simulink model "MSE452_Wind_Project_Model_Student_R2018b"  (R2023a)
settings: Solver=ode45  StartTime=0.0  StopTime=0.4  MaxStep=1e-5  RelTol=1e-3
values from neighbouring files (symbols this model uses):
  Cdc_wind = Cb_wind*3    [MSE452_Wind_Project_Model_Parameters_Student.m]
  Cin = 0.12*Cb_wind    [MSE452_Wind_Project_Model_Parameters_Student.m]
  Fb = 60    [MSE452_Wind_Project_Model_Parameters_Student.m]
  Fs_inv_wind = 3000    [MSE452_Wind_Project_Model_Parameters_Student.m]
  Fsampling = 10e3    (= 10000)    [MSE452_Wind_Project_Model_Parameters_Student.m]
  Ib_wind = Sb_wind/(3*Vb)    [MSE452_Wind_Project_Model_Parameters_Student.m]
  J = 2*H*Sb_wind/(Omega_gen_b^2)    (= 106.875544898)    [MSE452_Wind_Project_Model_Parameters_Student.m]
  Lboost_wind = 0.5*Lb_wind    [MSE452_Wind_Project_Model_Parameters_Student.m]
  Ld = 0.5*Lb_wind    [MSE452_Wind_Project_Model_Parameters_Student.m]
  Lgrid_pu_wind = 0.005    [MSE452_Wind_Project_Model_Parameters_Student.m]
  Lgrid_wind = 0.2*Lb_wind    [MSE452_Wind_Project_Model_Parameters_Student.m]
  Lq = 0.5*Lb_wind    [MSE452_Wind_Project_Model_Parameters_Student.m]
  Omega_gen_b = 2*pi*53.33    (= 335.082272432)    [MSE452_Wind_Project_Model_Parameters_Student.m]
  Ppairs = 16    [MSE452_Wind_Project_Model_Parameters_Student.m]
  Rgrid_wind = Rgrid_pu*Zb_wind    [MSE452_Wind_Project_Model_Parameters_Student.m]
  Rs = 0.01*Zb_wind    [MSE452_Wind_Project_Model_Parameters_Student.m]
  Tb = Ppairs*Sb_wind/Omega_gen_b    (= 71624.2009039)    [MSE452_Wind_Project_Model_Parameters_Student.m]
  Vb = 690/sqrt(3)    [MSE452_Wind_Project_Model_Parameters_Student.m]
  Vdc_ref_wind = sqrt(6)/ma    [MSE452_Wind_Project_Model_Parameters_Student.m]
  Wind_speed_b = 12    [MSE452_Wind_Project_Model_Parameters_Student.m]
undefined symbols (not defined in the file or in its folder): Rdc
libraries: spsCurrentMeasurementLib x11, spsVoltageMeasurementLib x8, spsSeriesRLCBranchLib x3, powerlib_extras x3, simulink x3, spsControlledVoltageSourceLib x2, spsUniversalBridgeLib x2, simulink_extras x2, spsThreePhaseSeriesRLCBranchLib x1, spsPermanentMagnetSynchronousMachineLib x1, spsPower3phInstantaneousLib x1, slpidlib x1
settings Model: Creator=Student  LastModifiedBy=auamai
settings SolverCC: ZeroCrossAlgorithm=Adaptive  AlgebraicLoopSolver=TrustRegion
settings DataIOCC: ReturnWorkspaceOutputs=off
settings OptimizationCC: LifeSpan=inf
settings DebuggingCC: UnconnectedInputMsg=warning  UnconnectedOutputMsg=warning  UnconnectedLineMsg=warning  ArithmeticOperatorsInVariantConditions=warning
settings HardwareCC: ProdBitPerSizeT=32  ProdBitPerPtrDiffT=32  ProdWordSize=32  ProdHWDeviceType=Specified
settings ModelReferenceCC: EnableRefExpFcnMdlSchedulingChecks=on
settings SFSimCC: SimUseLocalCustomCode=off  CustomCodeUndefinedFunction=UseInterfaceOnly
settings RTWCC: RTWUseLocalCustomCode=off
settings CodeAppCC: StateflowObjectComments=on
settings SimscapeCC: SimscapeNormalizeSystem=off

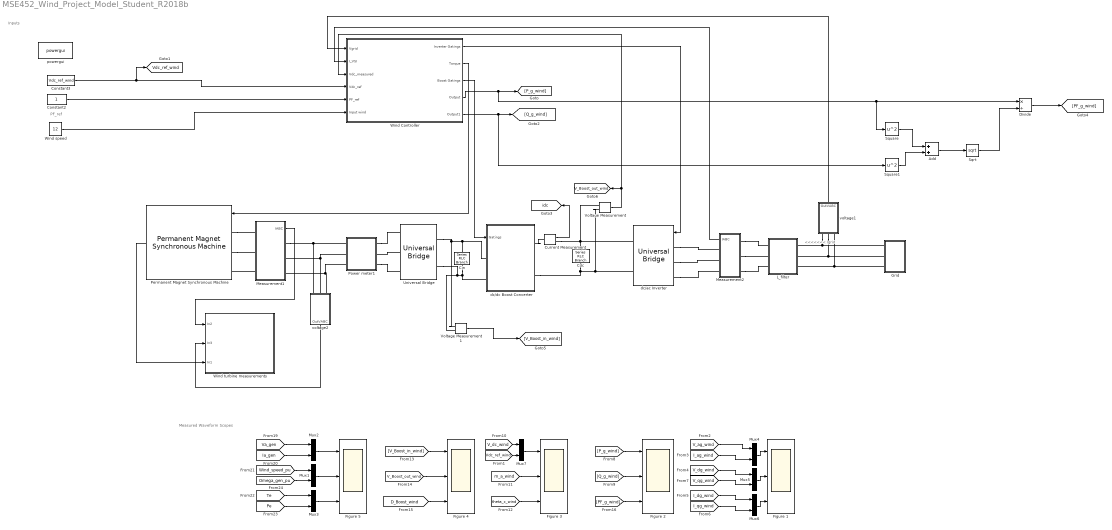
== system MSE452_Wind_Project_Model_Student_R2018b ==
  note: PF_ref
  note: Inputs
  note: <<<<<<< Igrid
  note: Measured Waveform Scopes
  " voltage1" : Subsystem  mask{Base=Vb}
      mask prompts: Base "Base value"
  " voltage2" : Subsystem  mask{Base=Vb}
      mask prompts: Base "Base value"
  Add : Sum
  Cdc : spsSeriesRLCBranchLib/Series RLC Branch  LConnTagsString=__new0  RConnTagsString=__new0  BranchType=C  Resistance=1e-4  Inductance=200e-6  SetiL0=off  InitialCurrent=0  Capacitance=Cdc_wind  Setx0=on  InitialVoltage=Vdc_capacitor_initial_wind  Measurements=None
  Cin : spsSeriesRLCBranchLib/Series RLC Branch  LConnTagsString=__new0  RConnTagsString=__new0  BranchType=C  Resistance=Rdc  Inductance=1e-3  SetiL0=off  InitialCurrent=0  Capacitance=Cin  Setx0=off  InitialVoltage=Vdc_capacitor_initial  Measurements=None
  Constant2 : Constant
  Constant3 : Constant  Value=Vdc_ref_wind
  Current Measurement : spsCurrentMeasurementLib/Current Measurement  PhasorSimulation=off  OutputType=Complex  PSBequivalent=0
  Divide : Product  Inputs=*/
  Figure {1..5} (5 alike) : Scope  NumInputPorts=3
  Grid : Subsystem
  L_filter : Subsystem
  Measurement1 : Subsystem  mask{Base=Ib_wind}
      mask prompts: Base "Base value"
  Measurement2 : Subsystem  mask{Base=Ib_wind}
      mask prompts: Base "Base value"
  Mux{1..7} (7 alike) : Mux  Inputs=2
  Permanent Magnet Synchronous Machine : spsPermanentMagnetSynchronousMachineLib/Permanent Magnet Synchronous Machine  NbPhases=3  FluxDistribution=Sinusoidal  RotorType=Salient-pole  MechanicalLoad=Torque Tm  PresetModel=No  ShowDetailedParameters=on  MeasurementBus=off  Resistance=Rs  Inductance=8.5e-3  dqInductances=[Ld, Lq]  La=0.000395  MachineConstant=Voltage Constant (V_peak L-L / krpm)  Flux=1.6813  VoltageCst=sqrt(2)*Vb*sqrt(3)*(1000/((Omega_gen_b/2/pi)*60/Ppairs))  TorqueCst=40.3518  Flat=120  Mechanical=[J 0.0004924 Ppairs 0]  PolePairs=4  InitialConditions=[15, 0, 0, 0]  InitialConditions5ph=[0 0 0 0 0 0]  RefAngle=Aligned with phase A axis (original Park)  IterativeDiscreteModel=Trapezoidal non iterative  TsBlock=-1  TsPowergui=0
  Power meter1 : Subsystem
  Sqrt : Sqrt
  Square : Math  Operator=square
  Square1 : Math  Operator=square
  Universal Bridge : spsUniversalBridgeLib/Universal Bridge  Arms=3  SnubberResistance=1e5  SnubberCapacitance=inf  Device=Diodes  Ron=1e-3  Lon=0  ForwardVoltages="[  0  0  ]"  ForwardVoltage=0  GTOparameters=[ 10e-6 , 20e-6 ]  IGBTparameters=[ 1e-6 , 2e-6 ]  Measurements=None  Measurements_2=None  converterType=Rectifier
  Voltage Measurement : spsVoltageMeasurementLib/Voltage Measurement  PhasorSimulation=off  OutputType=Complex  PSBequivalent=0
  Voltage Measurement1 : spsVoltageMeasurementLib/Voltage Measurement  PhasorSimulation=off  OutputType=Complex  PSBequivalent=0
  Wind Controller : Subsystem
  Wind speed : Constant  Value=12
  Wind turbine measurements : Subsystem
  dc/ac Inverter : spsUniversalBridgeLib/Universal Bridge  Arms=3  SnubberResistance=1e5  SnubberCapacitance=inf  Device=IGBT / Diodes  Ron=1e-6  Lon=0  ForwardVoltages="[  0  0  ]"  ForwardVoltage=0  GTOparameters=[ 10e-6 , 20e-6 ]  IGBTparameters=[ 1e-6 , 2e-6 ]  Measurements=None  Measurements_2=None  converterType=Rectifier
  dc/dc Boost Converter : Subsystem
  powergui : sps_lib/powergui  Priority=1  SimulationMode=Discrete  SampleTime=1e-6  frequency=60  Iterations=50  frequencyindice=0  Pbase=100e6  ErrMax=1e-4  UnitsV=kV  UnitsW=MW  buscounter=0  FunctionMessages=off  echomessages=off  EnableUseOfTLC=off  CurrentSourceSwitches=off  DisableSnubberDevices=off  DisableRonSwitches=off  DisableVfSwitches=off  DisplayEquations=off  AutomaticDiscreteSolvers=off  SolverType=Tustin/Backward Euler (TBE)  Interpol=off  ExternalGateDelay=off  methode=off  Ts=100  x0status=blocks  SPID=on  SwTol=0  HookPort=off  NonlinearTolerance=1e-4  nMaxIteration=100  ContinueOnMaxIteration=off  RestoreLinks=warning  ResistiveCurrentMeasurement=off  Frange=[0:2:500]  Ylog=off  Xlog=on  ShowGrid=off  save=off  variable=ZData  structure=0  ZoomFFT=off  StartTime=0.0  cycles=1  DisplayStyle=1  fundamental=60  FreqAxis=off  MaxFrequency=1000  frequencyindicesteady=1  RmsSteady=1  display=off
  tag scope: V_Boost_out_wind=global, Vdc_ref_wind=global, idc=global
  wires:
  [V_Boost_in_wind] -> Figure 4/1
  [Omega_gen_pu] -> Mux1/2
  [I_dg_wind] -> Mux6/1
  [Va_gen] -> Mux2/1
  Measurement2/1(IABC) -> Wind Controller/2(I_VSI)
  [Wind_speed_pu] -> Mux1/1
  [V_qg_wind] -> Mux5/2
  [m_a_wind] -> Figure 3/2
  [D_Boost_wind] -> Figure 4/3
  [V_Boost_out_wind] -> Figure 4/2
  Current Measurement/1 -> [idc]
  [I_ag_wind] -> Mux4/2
  Wind Controller/1(Inverter Gatings) -> dc/ac Inverter/1
  [Te] -> Mux3/1
  Voltage Measurement/1 -> Wind Controller/3(Vdc_measured), [V_Boost_out_wind]
  Voltage Measurement1/1 -> [V_Boost_in_wind]
  [V_dg_wind] -> Mux5/1
  " voltage1"/1(OutVABC) -> Wind Controller/1(Vgrid)
  [P_g_wind] -> Figure 2/1
  Mux2/1 -> Figure 5/1
  [theta_c_wind] -> Figure 3/3
  [Pe] -> Mux3/2
  [I_qg_wind] -> Mux6/2
  [Ia_gen] -> Mux2/2
  [V_ag_wind] -> Mux4/1
  [Q_g_wind] -> Figure 2/2
  [PF_g_wind] -> Figure 2/3
  Mux1/1 -> Figure 5/2
  Mux3/1 -> Figure 5/3
  Constant2/1 -> Wind Controller/5(PF_ref)
  Wind speed/1 -> Wind Controller/6(Input wind)
  Wind Controller/2(Torque) -> Permanent Magnet Synchronous Machine/1
  Permanent Magnet Synchronous Machine/1 -> Wind turbine measurements/3(In1)
  Measurement1/1(IABC) -> Wind turbine measurements/1(In2)
  " voltage2"/1(OutVABC) -> Wind turbine measurements/2(In3)
  Constant3/1 -> [Vdc_ref_wind], Wind Controller/4(Vdc_ref)
  Wind Controller/3(Boost Gatings) -> dc/dc Boost Converter/1(Gatings)
  Mux7/1 -> Figure 3/1
  [V_dc_wind] -> Mux7/1
  [Vdc_ref_wind] -> Mux7/2
  Wind Controller/4(Output) -> Square/1, Divide/1, [P_g_wind]
  Wind Controller/5(Output1) -> Square1/1, [Q_g_wind]
  Square/1 -> Add/1
  Square1/1 -> Add/2
  Add/1 -> Sqrt/1
  Sqrt/1 -> Divide/2
  Divide/1 -> [PF_g_wind]
  Mux6/1 -> Figure 1/3
  Mux5/1 -> Figure 1/2
  Mux4/1 -> Figure 1/1
  connections:
  dc/dc Boost Converter/LConn1 -- Voltage Measurement1/LConn1 -- Universal Bridge/RConn1 -- Cin/LConn1
  Cdc/LConn1 -- Current Measurement/RConn1 -- dc/ac Inverter/RConn1 -- Voltage Measurement/LConn1
  Voltage Measurement/LConn2 -- Cdc/RConn1 -- dc/dc Boost Converter/RConn2 -- dc/ac Inverter/RConn2
  Voltage Measurement1/LConn2 -- Universal Bridge/RConn2 -- Cin/RConn1 -- dc/dc Boost Converter/LConn2
  Measurement1/RConn1 -- Power meter1/LConn1 -- " voltage2"/LConn1
  " voltage2"/LConn3 -- Power meter1/LConn3 -- Measurement1/RConn3
  " voltage2"/LConn2 -- Power meter1/LConn2 -- Measurement1/RConn2
  Permanent Magnet Synchronous Machine/LConn1 -- Measurement1/LConn1
  Permanent Magnet Synchronous Machine/LConn2 -- Measurement1/LConn2
  Measurement2/LConn2 -- L_filter/RConn2
  dc/dc Boost Converter/RConn1 -- Current Measurement/LConn1
  dc/ac Inverter/LConn2 -- Measurement2/RConn2
  Measurement2/LConn1 -- L_filter/RConn1
  dc/ac Inverter/LConn1 -- Measurement2/RConn1
  Measurement2/LConn3 -- L_filter/RConn3
  Measurement1/LConn3 -- Permanent Magnet Synchronous Machine/LConn3
  dc/ac Inverter/LConn3 -- Measurement2/RConn3
  " voltage1"/LConn1 -- Grid/RConn1 -- L_filter/LConn1
  " voltage1"/LConn2 -- Grid/RConn2 -- L_filter/LConn2
  " voltage1"/LConn3 -- Grid/RConn3 -- L_filter/LConn3
  Power meter1/RConn1 -- Universal Bridge/LConn1
  Universal Bridge/LConn2 -- Power meter1/RConn2
  Power meter1/RConn3 -- Universal Bridge/LConn3

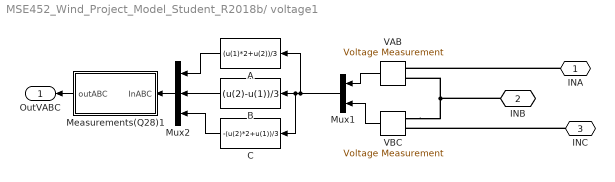
== system MSE452_Wind_Project_Model_Student_R2018b/ voltage1 ==
  A : Fcn  Expr=(u(1)*2+u(2))/3
  B : Fcn  Expr=(u(2)-u(1))/3
  C : Fcn  Expr=-(u(2)*2+u(1))/3
  Measurements(Q28)1 : Subsystem  mask{Base=Base}
      mask prompts: Base "Base Value"
  Mux1 : Mux  Inputs=2
  Mux2 : Mux  Inputs=3
  VAB : spsVoltageMeasurementLib/Voltage Measurement  PhasorSimulation=off  OutputType=Complex  PSBequivalent=0
  VBC : spsVoltageMeasurementLib/Voltage Measurement  PhasorSimulation=off  OutputType=Complex  PSBequivalent=0
  INA : PMIOPort  Side=Left
  INB : PMIOPort  Port=2  Side=Left
  INC : PMIOPort  Port=3  Side=Left
  OutVABC : Outport
  wires:
  Measurements(Q28)1/1(outABC) -> OutVABC/1
  VAB/1 -> Mux1/1
  VBC/1 -> Mux1/2
  Mux1/1 -> B/1, C/1, A/1
  A/1 -> Mux2/1
  B/1 -> Mux2/2
  Mux2/1 -> Measurements(Q28)1/1(InABC)
  C/1 -> Mux2/3
  connections:
  VBC/LConn1 -- VAB/LConn2 -- INB/RConn1
  INC/RConn1 -- VBC/LConn2
  INA/RConn1 -- VAB/LConn1

== system MSE452_Wind_Project_Model_Student_R2018b/ voltage2 ==
  A : Fcn  Expr=(u(1)*2+u(2))/3
  B : Fcn  Expr=(u(2)-u(1))/3
  C : Fcn  Expr=-(u(2)*2+u(1))/3
  Measurements(Q28)1 : Subsystem  mask{Base=Base}
      mask prompts: Base "Base Value"
  Mux1 : Mux  Inputs=2
  Mux2 : Mux  Inputs=3
  VAB : spsVoltageMeasurementLib/Voltage Measurement  PhasorSimulation=off  OutputType=Complex  PSBequivalent=0
  VBC : spsVoltageMeasurementLib/Voltage Measurement  PhasorSimulation=off  OutputType=Complex  PSBequivalent=0
  INA : PMIOPort  Side=Left
  INB : PMIOPort  Port=2  Side=Left
  INC : PMIOPort  Port=3  Side=Left
  OutVABC : Outport
  wires:
  C/1 -> Mux2/3
  Mux2/1 -> Measurements(Q28)1/1(InABC)
  B/1 -> Mux2/2
  A/1 -> Mux2/1
  Mux1/1 -> A/1, C/1, B/1
  VBC/1 -> Mux1/2
  VAB/1 -> Mux1/1
  Measurements(Q28)1/1(outABC) -> OutVABC/1
  connections:
  INA/RConn1 -- VAB/LConn1
  INC/RConn1 -- VBC/LConn2
  INB/RConn1 -- VAB/LConn2 -- VBC/LConn1

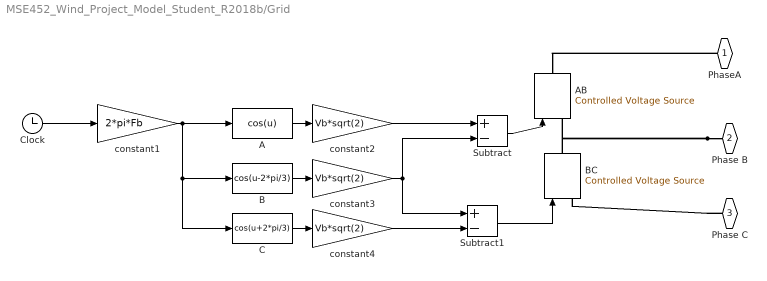
== system MSE452_Wind_Project_Model_Student_R2018b/Grid ==
  A : Fcn  Expr=cos(u)
  AB : spsControlledVoltageSourceLib/Controlled Voltage Source  Initialize=off  Source_Type=AC  Amplitude=0  Phase=0  Frequency=0  Measurements=None
  B : Fcn  Expr=cos(u-2*pi/3)
  BC : spsControlledVoltageSourceLib/Controlled Voltage Source  Initialize=off  Source_Type=AC  Amplitude=0  Phase=0  Frequency=0  Measurements=None
  C : Fcn  Expr=cos(u+2*pi/3)
  Clock : Clock
  Subtract : Sum  Inputs=+-
  Subtract1 : Sum  Inputs=+-
  constant1 : Gain  Gain=2*pi*Fb
  constant2 : Gain  Gain=Vb*sqrt(2)
  constant3 : Gain  Gain=Vb*sqrt(2)
  constant4 : Gain  Gain=Vb*sqrt(2)
  PhaseA : PMIOPort  Side=Right
  Phase B : PMIOPort  Port=2  Side=Right
  Phase C : PMIOPort  Port=3  Side=Right
  wires:
  Subtract/1 -> AB/1
  Subtract1/1 -> BC/1
  A/1 -> constant2/1
  B/1 -> constant3/1
  C/1 -> constant4/1
  Clock/1 -> constant1/1
  constant1/1 -> A/1, B/1, C/1
  constant2/1 -> Subtract/1
  constant3/1 -> Subtract/2, Subtract1/1
  constant4/1 -> Subtract1/2
  connections:
  Phase B/RConn1 -- BC/RConn1 -- AB/LConn1
  PhaseA/RConn1 -- AB/RConn1
  Phase C/RConn1 -- BC/LConn1

== system MSE452_Wind_Project_Model_Student_R2018b/L_filter ==
  Three-Phase Series RLC Branch1 : spsThreePhaseSeriesRLCBranchLib/Three-Phase Series RLC Branch  LConnTagsString=A|B|C  RConnTagsString=A|B|C  BranchType=RL  Resistance=Rgrid_wind  Inductance=Lgrid_wind  Capacitance=1e-6  Measurements=None
  In_A : PMIOPort  Side=Left
  out_A : PMIOPort  Port=2  Side=Right
  In_B : PMIOPort  Port=3  Side=Left
  out_B : PMIOPort  Port=4  Side=Right
  In_C : PMIOPort  Port=5  Side=Left
  out_C : PMIOPort  Port=6  Side=Right
  connections:
  In_B/RConn1 -- Three-Phase Series RLC Branch1/LConn2
  out_C/RConn1 -- Three-Phase Series RLC Branch1/RConn3
  out_B/RConn1 -- Three-Phase Series RLC Branch1/RConn2
  out_A/RConn1 -- Three-Phase Series RLC Branch1/RConn1
  Three-Phase Series RLC Branch1/LConn1 -- In_A/RConn1
  Three-Phase Series RLC Branch1/LConn3 -- In_C/RConn1

== system MSE452_Wind_Project_Model_Student_R2018b/Measurement1 ==
  IGA : spsCurrentMeasurementLib/Current Measurement  PhasorSimulation=off  OutputType=Complex  PSBequivalent=0
  IGB : spsCurrentMeasurementLib/Current Measurement  PhasorSimulation=off  OutputType=Complex  PSBequivalent=0
  IGC : spsCurrentMeasurementLib/Current Measurement  PhasorSimulation=off  OutputType=Complex  PSBequivalent=0
  Measurements(Q28)3 : Subsystem  mask{Base=Base}
      mask prompts: Base "Base Value"
  Mux1 : Mux  Inputs=3
  INA : PMIOPort  Side=Left
  outA : PMIOPort  Port=2  Side=Right
  INB : PMIOPort  Port=3  Side=Left
  outB : PMIOPort  Port=4  Side=Right
  INC : PMIOPort  Port=5  Side=Left
  outC : PMIOPort  Port=6  Side=Right
  IABC : Outport
  wires:
  IGC/1 -> Mux1/3
  IGB/1 -> Mux1/2
  IGA/1 -> Mux1/1
  Mux1/1 -> Measurements(Q28)3/1(InABC)
  Measurements(Q28)3/1(outABC) -> IABC/1
  connections:
  INA/RConn1 -- IGA/LConn1
  outA/RConn1 -- IGA/RConn1
  INB/RConn1 -- IGB/LConn1
  outB/RConn1 -- IGB/RConn1
  INC/RConn1 -- IGC/LConn1
  outC/RConn1 -- IGC/RConn1

== system MSE452_Wind_Project_Model_Student_R2018b/Measurement2 ==
  IGA : spsCurrentMeasurementLib/Current Measurement  PhasorSimulation=off  OutputType=Complex  PSBequivalent=0
  IGB : spsCurrentMeasurementLib/Current Measurement  PhasorSimulation=off  OutputType=Complex  PSBequivalent=0
  IGC : spsCurrentMeasurementLib/Current Measurement  PhasorSimulation=off  OutputType=Complex  PSBequivalent=0
  Measurements(Q28)3 : Subsystem  mask{Base=Base}
      mask prompts: Base "Base Value"
  Mux1 : Mux  Inputs=3
  INA : PMIOPort  Side=Left
  outA : PMIOPort  Port=2  Side=Right
  INB : PMIOPort  Port=3  Side=Left
  outB : PMIOPort  Port=4  Side=Right
  INC : PMIOPort  Port=5  Side=Left
  outC : PMIOPort  Port=6  Side=Right
  IABC : Outport
  wires:
  Measurements(Q28)3/1(outABC) -> IABC/1
  Mux1/1 -> Measurements(Q28)3/1(InABC)
  IGA/1 -> Mux1/1
  IGB/1 -> Mux1/2
  IGC/1 -> Mux1/3
  connections:
  outC/RConn1 -- IGC/RConn1
  INC/RConn1 -- IGC/LConn1
  outB/RConn1 -- IGB/RConn1
  INB/RConn1 -- IGB/LConn1
  outA/RConn1 -- IGA/RConn1
  INA/RConn1 -- IGA/LConn1

== system MSE452_Wind_Project_Model_Student_R2018b/Power meter1 ==
  1st order filter1 : Subsystem  mask{F0=10, Fs=Fsampling}
      mask prompts: F0 "Cut off Frequency"; Fs "Sampling Frequency"
  1st order filter2 : Subsystem  mask{F0=10, Fs=Fsampling}
      mask prompts: F0 "Cut off Frequency"; Fs "Sampling Frequency"
  "Power (3ph, Instantaneous)1" : spsPower3phInstantaneousLib/Power (3ph, Instantaneous)
  Scope2 : Scope  NumInputPorts=2
  Scope3 : Scope  NumInputPorts=2
  meter1 : Subsystem  mask{Base=1}
      mask prompts: Base "Base value"
  A_in1 : PMIOPort  Side=Left
  B_in1 : PMIOPort  Port=2  Side=Left
  C_in1 : PMIOPort  Port=3  Side=Left
  A_out1 : PMIOPort  Port=4  Side=Right
  B_out1 : PMIOPort  Port=5  Side=Right
  C_out1 : PMIOPort  Port=6  Side=Right
  wires:
  "Power (3ph, Instantaneous)1"/2 -> 1st order filter2/1(in)
  1st order filter1/1(Out) -> Scope3/1
  meter1/2(VABC) -> Scope2/1, "Power (3ph, Instantaneous)1"/1
  "Power (3ph, Instantaneous)1"/1 -> 1st order filter1/1(in)
  1st order filter2/1(Out) -> Scope3/2
  meter1/1(IABC) -> Scope2/2, "Power (3ph, Instantaneous)1"/2
  connections:
  B_in1/RConn1 -- meter1/RConn2
  meter1/LConn3 -- C_out1/RConn1
  B_out1/RConn1 -- meter1/LConn2
  C_in1/RConn1 -- meter1/RConn3
  meter1/LConn1 -- A_out1/RConn1
  A_in1/RConn1 -- meter1/RConn1

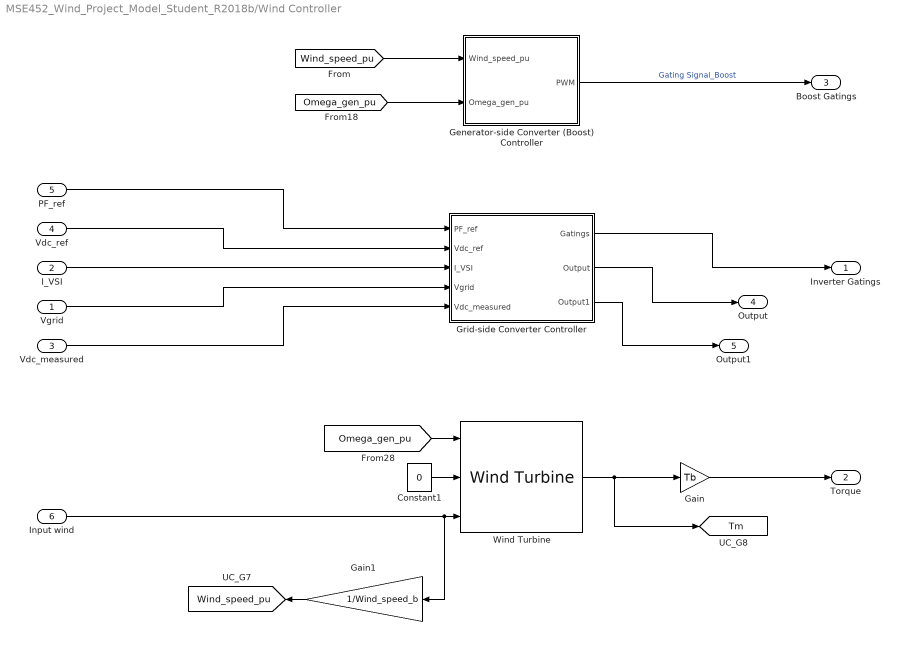
== system MSE452_Wind_Project_Model_Student_R2018b/Wind Controller ==
  Vgrid : Inport
  I_VSI : Inport  Port=2
  Vdc_measured : Inport  Port=3
  Vdc_ref : Inport  Port=4
  PF_ref : Inport  Port=5
  Input wind : Inport  Port=6
  Constant1 : Constant  Value=0
  Gain : Gain  Gain=Tb
  Gain1 : Gain  Gain=1/Wind_speed_b
  Generator-side Converter (Boost) Controller : Subsystem
  Grid-side Converter Controller : Subsystem
  Wind Turbine : spsWindTurbineLib/Wind Turbine  Pnom=Sb_wind  Pelec_base=Sb_wind  wind_base=Wind_speed_b  P_wind_base=1  speed_nom=1  pitch_angle=0  c1_c6="[0.51763          116          0.4            5           21     0.006795]"  cp_nom=0.48  lambda_nom=8.1
  Inverter Gatings : Outport
  Torque : Outport  Port=2
  Boost Gatings : Outport  Port=3
  Output : Outport  Port=4
  Output1 : Outport  Port=5
  tag scope: Tm=global, Wind_speed_pu=global
  wires:
  Vdc_measured/1 -> Grid-side Converter Controller/5(Vdc_measured)
  Vgrid/1 -> Grid-side Converter Controller/4(Vgrid)
  Grid-side Converter Controller/1(Gatings) -> Inverter Gatings/1
  PF_ref/1 -> Grid-side Converter Controller/1(PF_ref)
  I_VSI/1 -> Grid-side Converter Controller/3(I_VSI)
  Vdc_ref/1 -> Grid-side Converter Controller/2(Vdc_ref)
  [Wind_speed_pu] -> Generator-side Converter (Boost) Controller/1(Wind_speed_pu)
  [Omega_gen_pu] -> Generator-side Converter (Boost) Controller/2(Omega_gen_pu)
  Generator-side Converter (Boost) Controller/1(PWM) -> Boost Gatings/1  "Gating Signal_Boost"
  [Omega_gen_pu] -> Wind Turbine/1
  Wind Turbine/1 -> [Tm], Gain/1
  Input wind/1 -> Gain1/1, Wind Turbine/3
  Constant1/1 -> Wind Turbine/2
  Gain/1 -> Torque/1
  Gain1/1 -> [Wind_speed_pu]
  Grid-side Converter Controller/2(Output) -> Output/1
  Grid-side Converter Controller/3(Output1) -> Output1/1

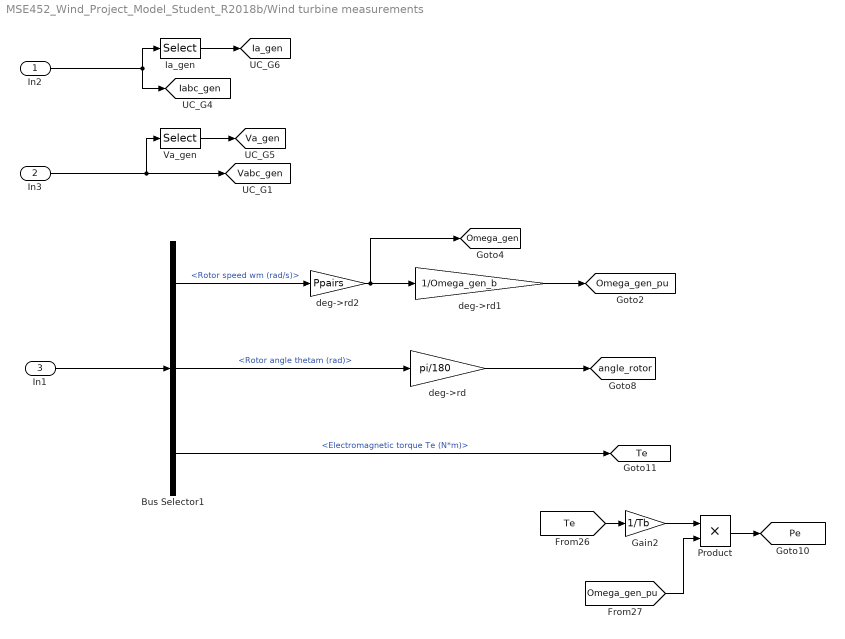
== system MSE452_Wind_Project_Model_Student_R2018b/Wind turbine measurements ==
  In2 : Inport
  In3 : Inport  Port=2
  In1 : Inport  Port=3
  Bus Selector1 : BusSelector  OutputSignals=Rotor speed wm (rad/s),Rotor angle thetam (rad),Electromagnetic torque Te (N*m)
  Gain2 : Gain  Gain=1/Tb
  Ia_gen : Selector  InputPortWidth=3  IndexOptions=Index vector (dialog)  Indices=1  OutputSizes=1
  Product : Product
  Va_gen : Selector  InputPortWidth=3  IndexOptions=Index vector (dialog)  Indices=1  OutputSizes=1
  deg->rd : Gain  Gain=pi/180  SaturateOnIntegerOverflow=on  OutDataTypeStr=Inherit: Same as input  ParamDataTypeStr=Inherit: Same as input
  deg->rd1 : Gain  Gain=1/Omega_gen_b  SaturateOnIntegerOverflow=on  OutDataTypeStr=Inherit: Same as input  ParamDataTypeStr=Inherit: Same as input
  deg->rd2 : Gain  Gain=Ppairs  SaturateOnIntegerOverflow=on  OutDataTypeStr=Inherit: Same as input  ParamDataTypeStr=Inherit: Same as input
  tag scope: Ia_gen=global, Iabc_gen=global, Omega_gen=global, Omega_gen_pu=global, Pe=global, Te=global, Va_gen=global, Vabc_gen=global, angle_rotor=global
  wires:
  In1/1 -> Bus Selector1/1
  deg->rd2/1 -> deg->rd1/1, [Omega_gen]
  deg->rd/1 -> [angle_rotor]
  deg->rd1/1 -> [Omega_gen_pu]
  Bus Selector1/1 -> deg->rd2/1  "<Rotor speed wm (rad/s)>"
  Bus Selector1/3 -> [Te]  "<Electromagnetic torque Te (N*m)>"
  Bus Selector1/2 -> deg->rd/1  "<Rotor angle thetam (rad)>"
  [Omega_gen_pu] -> Product/2
  Product/1 -> [Pe]
  Gain2/1 -> Product/1
  [Te] -> Gain2/1
  Va_gen/1 -> [Va_gen]
  In3/1 -> [Vabc_gen], Va_gen/1
  In2/1 -> [Iabc_gen], Ia_gen/1
  Ia_gen/1 -> [Ia_gen]

== system MSE452_Wind_Project_Model_Student_R2018b/dc//dc Boost Converter ==
  Gatings : Inport
  Current Measurement : spsCurrentMeasurementLib/Current Measurement  PhasorSimulation=off  OutputType=Complex  PSBequivalent=0
  Diode1 : spsDiodeLib/Diode  Ron=1e-3  Lon=0  Vf=0  IC=0  UseSnubber=off  Rs=inf  Cs=inf  Measurements=off
  L : spsSeriesRLCBranchLib/Series RLC Branch  LConnTagsString=__new0  RConnTagsString=__new0  BranchType=L  Resistance=0.01  Inductance=Lboost_wind  SetiL0=off  InitialCurrent=0  Capacitance=1e-6  Setx0=off  InitialVoltage=0  Measurements=None
  Mosfet : spsMosfetLib/Mosfet  Ron=0.001  Lon=0  Rd=0.01  Vfd=0  IC=0  Rs=1e5  Cs=inf  Measurements=off
  Scope : Scope
  In + : PMIOPort  Side=Left
  In - : PMIOPort  Port=2  Side=Left
  Out + : PMIOPort  Port=3  Side=Right
  Out - : PMIOPort  Port=4  Side=Right
  wires:
  Current Measurement/1 -> Scope/1
  Gatings/1 -> Mosfet/1  "Boost Gating Signal"
  connections:
  Current Measurement/LConn1 -- In +/RConn1
  Current Measurement/RConn1 -- L/LConn1
  Mosfet/LConn1 -- L/RConn1 -- Diode1/LConn1
  Diode1/RConn1 -- Out +/RConn1
  Mosfet/RConn1 -- In -/RConn1 -- Out -/RConn1

== system MSE452_Wind_Project_Model_Student_R2018b/ voltage1/Measurements(Q28)1 ==
  InABC : Inport
  Demux : Demux  Outputs=3
  Gain1 : Gain  Gain=1/Base
  Gain2 : Gain  Gain=1/Base
  Gain3 : Gain  Gain=1/Base
  Mux : Mux  Inputs=3
  outABC : Outport
  wires:
  Mux/1 -> outABC/1
  Demux/1 -> Gain2/1
  InABC/1 -> Demux/1
  Gain2/1 -> Mux/1
  Gain1/1 -> Mux/2
  Gain3/1 -> Mux/3
  Demux/2 -> Gain1/1
  Demux/3 -> Gain3/1

== system MSE452_Wind_Project_Model_Student_R2018b/ voltage2/Measurements(Q28)1 ==
  InABC : Inport
  Demux : Demux  Outputs=3
  Gain1 : Gain  Gain=1/Base
  Gain2 : Gain  Gain=1/Base
  Gain3 : Gain  Gain=1/Base
  Mux : Mux  Inputs=3
  outABC : Outport
  wires:
  Demux/3 -> Gain3/1
  Demux/2 -> Gain1/1
  Gain3/1 -> Mux/3
  Gain1/1 -> Mux/2
  Gain2/1 -> Mux/1
  InABC/1 -> Demux/1
  Demux/1 -> Gain2/1
  Mux/1 -> outABC/1

== system MSE452_Wind_Project_Model_Student_R2018b/Measurement1/Measurements(Q28)3 ==
  InABC : Inport
  Demux : Demux  Outputs=3
  Gain1 : Gain  Gain=1/Base
  Gain2 : Gain  Gain=1/Base
  Gain3 : Gain  Gain=1/Base
  Mux : Mux  Inputs=3
  outABC : Outport
  wires:
  Demux/3 -> Gain3/1
  Demux/2 -> Gain1/1
  Gain3/1 -> Mux/3
  Gain1/1 -> Mux/2
  Gain2/1 -> Mux/1
  InABC/1 -> Demux/1
  Demux/1 -> Gain2/1
  Mux/1 -> outABC/1

== system MSE452_Wind_Project_Model_Student_R2018b/Measurement2/Measurements(Q28)3 ==
  InABC : Inport
  Demux : Demux  Outputs=3
  Gain1 : Gain  Gain=1/Base
  Gain2 : Gain  Gain=1/Base
  Gain3 : Gain  Gain=1/Base
  Mux : Mux  Inputs=3
  outABC : Outport
  wires:
  Mux/1 -> outABC/1
  Demux/1 -> Gain2/1
  InABC/1 -> Demux/1
  Gain2/1 -> Mux/1
  Gain1/1 -> Mux/2
  Gain3/1 -> Mux/3
  Demux/2 -> Gain1/1
  Demux/3 -> Gain3/1

== system MSE452_Wind_Project_Model_Student_R2018b/Power meter1/1st order filter1 ==
  in : Inport
  Discrete Transfer 1Hz3 : DiscreteTransferFcn  Numerator=[1/Fs*(2*pi*F0) 1/Fs*(2*pi*F0) ]  Denominator="[((2*pi*F0)/Fs+2)  ((2*pi*F0)/Fs-2)]"  SampleTime=1/Fs
  Out : Outport
  wires:
  in/1 -> Discrete Transfer 1Hz3/1
  Discrete Transfer 1Hz3/1 -> Out/1

== system MSE452_Wind_Project_Model_Student_R2018b/Power meter1/1st order filter2 ==
  in : Inport
  Discrete Transfer 1Hz3 : DiscreteTransferFcn  Numerator=[1/Fs*(2*pi*F0) 1/Fs*(2*pi*F0) ]  Denominator="[((2*pi*F0)/Fs+2)  ((2*pi*F0)/Fs-2)]"  SampleTime=1/Fs
  Out : Outport
  wires:
  in/1 -> Discrete Transfer 1Hz3/1
  Discrete Transfer 1Hz3/1 -> Out/1

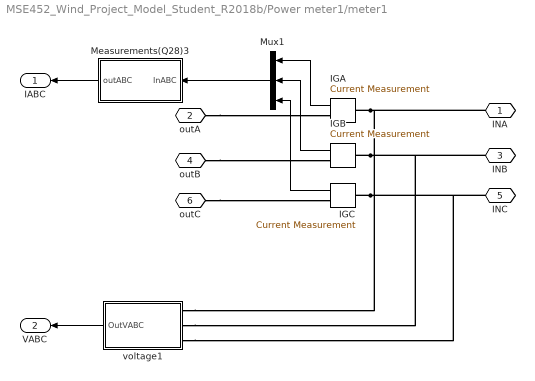
== system MSE452_Wind_Project_Model_Student_R2018b/Power meter1/meter1 ==
  " voltage1" : Subsystem  mask{Base=1}
      mask prompts: Base "Base value"
  IGA : spsCurrentMeasurementLib/Current Measurement  PhasorSimulation=off  OutputType=Complex  PSBequivalent=0
  IGB : spsCurrentMeasurementLib/Current Measurement  PhasorSimulation=off  OutputType=Complex  PSBequivalent=0
  IGC : spsCurrentMeasurementLib/Current Measurement  PhasorSimulation=off  OutputType=Complex  PSBequivalent=0
  Measurements(Q28)3 : Subsystem  mask{Base=1}
      mask prompts: Base "Base Value"
  Mux1 : Mux  Inputs=3
  INA : PMIOPort  Side=Left
  outA : PMIOPort  Port=2  Side=Right
  INB : PMIOPort  Port=3  Side=Left
  outB : PMIOPort  Port=4  Side=Right
  INC : PMIOPort  Port=5  Side=Left
  outC : PMIOPort  Port=6  Side=Right
  IABC : Outport  VectorParamsAs1DForOutWhenUnconnected=off
  VABC : Outport  Port=2  VectorParamsAs1DForOutWhenUnconnected=off
  wires:
  Measurements(Q28)3/1(outABC) -> IABC/1
  Mux1/1 -> Measurements(Q28)3/1(InABC)
  IGA/1 -> Mux1/1
  IGB/1 -> Mux1/2
  IGC/1 -> Mux1/3
  " voltage1"/1(OutVABC) -> VABC/1
  connections:
  outC/RConn1 -- IGC/RConn1
  IGC/LConn1 -- INC/RConn1 -- " voltage1"/LConn3
  outB/RConn1 -- IGB/RConn1
  IGB/LConn1 -- INB/RConn1 -- " voltage1"/LConn2
  outA/RConn1 -- IGA/RConn1
  IGA/LConn1 -- INA/RConn1 -- " voltage1"/LConn1

== system MSE452_Wind_Project_Model_Student_R2018b/Wind Controller/Generator-side Converter (Boost) Controller ==
  Wind_speed_pu : Inport
  Omega_gen_pu : Inport  Port=2
  PID Controller : slpidlib/PID Controller  Controller=PI  Form=Parallel  TimeDomain=Continuous-time  UseExternalTs=off  SampleTime=-1  IntegratorMethod=Forward Euler  FilterMethod=Forward Euler  ControllerParametersSource=internal  P=-25  I=-30  UseKiTs=off  D=0  N=100  UseFilter=on  TunerSelectOption=Transfer Function Based (PID Tuner App)  InitialConditionSource=internal  InitialConditionForIntegrator=0  InitialConditionForFilter=0  DifferentiatorICPrevScaledInput=0  ExternalReset=none  TrackingMode=off  Kt=1  LimitOutput=on  SatLimitsSource=internal  UpperSaturationLimit=2  LowerSaturationLimit=-2  LinearizeAsGain=on  AntiWindupMode=clamping  Kb=1  LimitIntegrator=off  UpperIntegratorSaturationLimit=inf  LowerIntegratorSaturationLimit=-inf  POutMin=[]  POutMax=[]  IOutMin=[]  IOutMax=[]  DOutMin=[]  DOutMax=[]  NOutMin=[]  NOutMax=[]  SumOutMin=[]  SumOutMax=[]  SaturationOutMin=[]  SaturationOutMax=[]  PParamMin=[]  PParamMax=[]  IParamMin=[]  IParamMax=[]  DParamMin=[]  DParamMax=[]  NParamMin=[]  NParamMax=[]  KbParamMin=[]  KbParamMax=[]  KtParamMin=[]  KtParamMax=[]  KbOutMin=[]  KbOutMax=[]  KtOutMin=[]  KtOutMax=[]  IntegratorOutMin=[]  IntegratorOutMax=[]  FilterOutMin=[]  FilterOutMax=[]  SumI1OutMin=[]  SumI1OutMax=[]  SumI2OutMin=[]  SumI2OutMax=[]  SumI3OutMin=[]  SumI3OutMax=[]  SumI4OutMin=[]  SumI4OutMax=[]  SumDOutMin=[]  SumDOutMax=[]  DifferentiatorOutMin=[]  DifferentiatorOutMax=[]  FilterDiffOutCoefMin=[]  FilterDiffOutCoefMax=[]  ReciprocalOutMin=[]  ReciprocalOutMax=[]  SumDenOutMin=[]  SumDenOutMax=[]  SumNumOutMin=[]  SumNumOutMax=[]  DivideOutMin=[]  DivideOutMax=[]  UdiffTsProdOutMin=[]  UdiffTsProdOutMax=[]  NTsProdOutMin=[]  NTsProdOutMax=[]  UintegralTsProdOutMin=[]  UintegralTsProdOutMax=[]  UngainTsProdOutMin=[]  UngainTsProdOutMax=[]  ClampingZeroOutDataTypeStr=Inherit: Inherit via back propagation  ClampingZeroOutMin=[]  ClampingZeroOutMax=[]  FilterDenConstantOutDataTypeStr=Inherit: Inherit via back propagation  FilterDenConstantOutMin=[]  FilterDenConstantOutMax=[]  PCopyOutDataTypeStr=Inherit: Inherit via back propagation  PCopyOutMin=[]  PCopyOutMax=[]  NCopyOutDataTypeStr=Inherit: Inherit via back propagation  NCopyOutMin=[]  NCopyOutMax=[]  IntegratorContinuousStateAttributes=''  IntegratorStateMustResolveToSignalObject=off  IntegratorRTWStateStorageClass=Auto  FilterContinuousStateAttributes=''  FilterStateMustResolveToSignalObject=off  FilterRTWStateStorageClass=Auto  ParallelPVariant=InternalParameters  IdealPVariant=Disabled  IVariant=InternalParameters  DVariant=Disabled  IntegratorVariant=Continuous  SatVariant=Enabled  AWVariant=ContClampingParallel  PCopyVariant=Disabled  TRVariant=Disabled  FdbkBlocksVariant=Forward  IdealPFdbkVariant=Disabled  SatFdbkVariant=Disabled  DerivativeFilterVariant=Disabled  NVariant=Disabled  NCopyVariant=Disabled_SignalSpec  FilterICVariant=Disabled  IntegratorICVariant=InternalICs  ExternalResetVariant=Disabled  TRSumVariant=Passthrough  SumFdbkVariant=Disabled  SumVariant=Sum_PI  TsampFilterVariant=InternalTs  TsampNgainVariant=Passthrough  TsampIntegralVariant=Disabled_SignalSpec  ExternalSaturationOutDataTypeStr=Inherit: Same as second input
  PWM Generator (DC-DC) : spsPWMGeneratorDCDCLib/PWM Generator (DC-DC)  Fsw=Fs_boost_wind  Ts=0
  Saturation : Saturate  UpperLimit=1  LowerLimit=0
  Scope2 : Scope  NumInputPorts=2
  Sum1 : Sum  Inputs=|+-
  PWM : Outport
  tag scope: D_Boost_wind=global
  wires:
  Sum1/1 -> Scope2/1, PID Controller/1
  PWM Generator (DC-DC)/1 -> Scope2/2, PWM/1
  PID Controller/1 -> Saturation/1
  Saturation/1 -> [D_Boost_wind], PWM Generator (DC-DC)/1
  Wind_speed_pu/1 -> Sum1/1  "Wind_speed_pu"
  Omega_gen_pu/1 -> Sum1/2  "Omega_gen_pu"

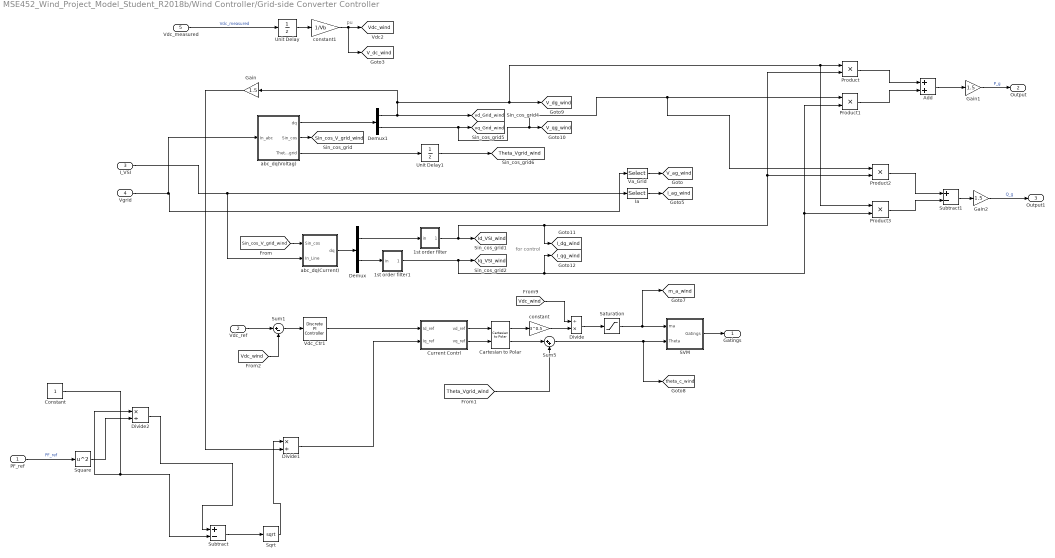
== system MSE452_Wind_Project_Model_Student_R2018b/Wind Controller/Grid-side Converter Controller ==
  note: for control
  note: pu
  PF_ref : Inport
  Vdc_ref : Inport  Port=2
  I_VSI : Inport  Port=3
  Vgrid : Inport  Port=4
  Vdc_measured : Inport  Port=5
  1st order filter : Subsystem  mask{F0=500, Fs=Fsampling}
      mask prompts: F0 "Cut off Frequency"; Fs "Sampling Frequency"
  1st order filter1 : Subsystem  mask{F0=500, Fs=Fsampling}
      mask prompts: F0 "Cut off Frequency"; Fs "Sampling Frequency"
  Add : Sum
  Cartesian to Polar : simulink_extras/Transformations/Cartesian to Polar
  Constant : Constant
  Current Contrl : Subsystem
  Demux : Demux  Outputs=2
  Demux1 : Demux  Outputs=2
  Divide : Product  Inputs=/*
  Divide1 : Product  Inputs=*/
  Divide2 : Product  Inputs=*/
  Gain : Gain  Gain=1.5
  Gain1 : Gain  Gain=1.5
  Gain2 : Gain  Gain=1.5
  Ia : Selector  InputPortWidth=3  IndexOptions=Index vector (dialog)  Indices=1  OutputSizes=1
  Product{,1..3} (4 alike) : Product
  SVM : Subsystem  mask{Fs=Fs_inv_wind}
      mask prompts: Fs "Switching frequency"
  Saturation : Saturate  UpperLimit=1  LowerLimit=0  SampleTime=1/Fsampling
  Sqrt : Sqrt
  Square : Math  Operator=square
  Subtract : Sum  Inputs=+-
  Subtract1 : Sum  Inputs=+-
  Sum1 : Sum  Inputs=|+-
  Sum5 : Sum  Inputs=|++
  Unit Delay : UnitDelay  InitialCondition=Vb*3^0.5  SampleTime=1/Fsampling  HasFrameUpgradeWarning=on
  Unit Delay1 : UnitDelay  InitialCondition=Vb*3^0.5  SampleTime=1/Fsampling  HasFrameUpgradeWarning=on
  Va_Grid : Selector  InputPortWidth=3  IndexOptions=Index vector (dialog)  Indices=1  OutputSizes=1
  Vdc_Ctr1 : powerlib_extras/Discrete  Control Blocks/Discrete PI Controller  Kp=1.0  Ki=200  Par_Limits=[1.5 -1.5]  Init=0  Ts=1/Fsampling
  abc_dq(Current) : Subsystem
  abc_dq(Voltag) : Subsystem
  constant : Gain  Gain=3^0.5
  constant1 : Gain  Gain=1/Vb
  Gatings : Outport
  Output : Outport  Port=2
  Output1 : Outport  Port=3
  tag scope: I_ag_wind=global, I_dg_wind=global, I_qg_wind=global, Id_VSI_wind=global, Iq_VSI_wind=global, Sin_cos_V_grid_wind=global, Theta_Vgrid_wind=global, V_ag_wind=global, V_dc_wind=global, V_dg_wind=global, V_qg_wind=global, Vdc_wind=global, m_a_wind=global, theta_c_wind=global, vd_Grid_wind=global, vq_Grid_wind=global
  wires:
  abc_dq(Current)/1(dq) -> Demux/1
  abc_dq(Voltag)/1(dq) -> Demux1/1
  abc_dq(Voltag)/2(Sin_cos) -> [Sin_cos_V_grid_wind]
  [Sin_cos_V_grid_wind] -> abc_dq(Current)/1(Sin_cos)
  Demux/1 -> 1st order filter/1(in)
  Demux/2 -> 1st order filter1/1(in)
  abc_dq(Voltag)/3(Theta_Vgrid) -> Unit Delay1/1
  Cartesian to Polar/1 -> constant/1
  Cartesian to Polar/2 -> Sum5/1
  Current Contrl/1(vd_ref) -> Cartesian to Polar/1
  Current Contrl/2(vq_ref) -> Cartesian to Polar/2
  [Vdc_wind] -> Divide/1
  constant/1 -> Divide/2
  Divide/1 -> Saturation/1
  [Vdc_wind] -> Sum1/2
  Sum1/1 -> Vdc_Ctr1/1
  SVM/1(Gatings) -> Gatings/1
  Unit Delay/1 -> constant1/1
  [Theta_Vgrid_wind] -> Sum5/2
  Unit Delay1/1 -> [Theta_Vgrid_wind]
  Demux1/1 -> [vd_Grid_wind], Gain/1, Product3/1, Product/1, [V_dg_wind]
  Demux1/2 -> Product2/1, Product1/1, [V_qg_wind], [vq_Grid_wind]
  Va_Grid/1 -> [V_ag_wind]
  Ia/1 -> [I_ag_wind]
  1st order filter/1(Out) -> Product2/2, Product/2, [I_dg_wind], [Id_VSI_wind]
  1st order filter1/1(Out) -> Product3/2, Product1/2, [I_qg_wind], [Iq_VSI_wind]
  constant1/1 -> [V_dc_wind], [Vdc_wind]
  Vdc_Ctr1/1 -> Current Contrl/1(Id_ref)
  Sum5/1 -> [theta_c_wind], SVM/2(Theta)
  Saturation/1 -> [m_a_wind], SVM/1(ma)
  I_VSI/1 -> abc_dq(Current)/2(In_Line), Ia/1
  Vgrid/1 -> abc_dq(Voltag)/1(In_abc), Va_Grid/1
  Constant/1 -> Subtract/2, Divide2/1
  Square/1 -> Divide2/2
  Divide2/1 -> Subtract/1
  Subtract/1 -> Sqrt/1
  Sqrt/1 -> Divide1/1
  PF_ref/1 -> Square/1  "PF_ref"
  Gain/1 -> Divide1/2
  Vdc_ref/1 -> Sum1/1
  Vdc_measured/1 -> Unit Delay/1  "Vdc_measured"
  Product/1 -> Add/1
  Product1/1 -> Add/2
  Add/1 -> Gain1/1
  Product2/1 -> Subtract1/1
  Product3/1 -> Subtract1/2
  Subtract1/1 -> Gain2/1
  Gain1/1 -> Output/1  "P_g"
  Gain2/1 -> Output1/1  "Q_g"
  Divide1/1 -> Current Contrl/2(Iq_ref)

== system MSE452_Wind_Project_Model_Student_R2018b/Power meter1/meter1/ voltage1 ==
  A : Fcn  Expr=(u(1)*2+u(2))/3
  B : Fcn  Expr=(u(2)-u(1))/3
  C : Fcn  Expr=-(u(2)*2+u(1))/3
  Measurements(Q28)1 : Subsystem  mask{Base=Base}
      mask prompts: Base "Base Value"
  Mux1 : Mux  Inputs=2
  Mux2 : Mux  Inputs=3
  VAB : spsVoltageMeasurementLib/Voltage Measurement  PhasorSimulation=off  OutputType=Complex  PSBequivalent=0
  VBC : spsVoltageMeasurementLib/Voltage Measurement  PhasorSimulation=off  OutputType=Complex  PSBequivalent=0
  INA : PMIOPort  Side=Left
  INB : PMIOPort  Port=2  Side=Left
  INC : PMIOPort  Port=3  Side=Left
  OutVABC : Outport  VectorParamsAs1DForOutWhenUnconnected=off
  wires:
  Measurements(Q28)1/1(outABC) -> OutVABC/1
  VAB/1 -> Mux1/1
  VBC/1 -> Mux1/2
  Mux1/1 -> B/1, C/1, A/1
  A/1 -> Mux2/1
  B/1 -> Mux2/2
  Mux2/1 -> Measurements(Q28)1/1(InABC)
  C/1 -> Mux2/3
  connections:
  VBC/LConn1 -- VAB/LConn2 -- INB/RConn1
  INC/RConn1 -- VBC/LConn2
  INA/RConn1 -- VAB/LConn1

== system MSE452_Wind_Project_Model_Student_R2018b/Power meter1/meter1/Measurements(Q28)3 ==
  InABC : Inport
  Demux : Demux  Outputs=3
  Gain1 : Gain  Gain=1/Base
  Gain2 : Gain  Gain=1/Base
  Gain3 : Gain  Gain=1/Base
  Mux : Mux  Inputs=3
  outABC : Outport  VectorParamsAs1DForOutWhenUnconnected=off
  wires:
  Mux/1 -> outABC/1
  Demux/1 -> Gain2/1
  InABC/1 -> Demux/1
  Gain2/1 -> Mux/1
  Gain1/1 -> Mux/2
  Gain3/1 -> Mux/3
  Demux/2 -> Gain1/1
  Demux/3 -> Gain3/1

== system MSE452_Wind_Project_Model_Student_R2018b/Wind Controller/Grid-side Converter Controller/1st order filter ==
  in : Inport
  Discrete Transfer 1Hz3 : DiscreteTransferFcn  Numerator=[1/Fs*(2*pi*F0) 1/Fs*(2*pi*F0) ]  Denominator="[((2*pi*F0)/Fs+2)  ((2*pi*F0)/Fs-2)]"  SampleTime=1/Fs
  Out : Outport
  wires:
  Discrete Transfer 1Hz3/1 -> Out/1
  in/1 -> Discrete Transfer 1Hz3/1

== system MSE452_Wind_Project_Model_Student_R2018b/Wind Controller/Grid-side Converter Controller/1st order filter1 ==
  in : Inport
  Discrete Transfer 1Hz3 : DiscreteTransferFcn  Numerator=[1/Fs*(2*pi*F0) 1/Fs*(2*pi*F0) ]  Denominator="[((2*pi*F0)/Fs+2)  ((2*pi*F0)/Fs-2)]"  SampleTime=1/Fs
  Out : Outport
  wires:
  in/1 -> Discrete Transfer 1Hz3/1
  Discrete Transfer 1Hz3/1 -> Out/1

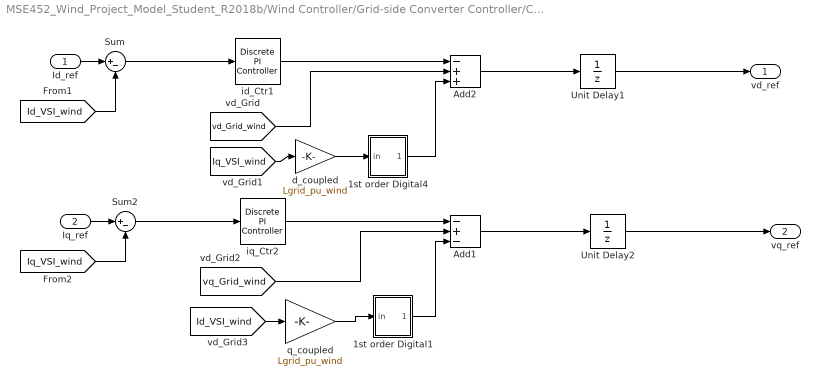
== system MSE452_Wind_Project_Model_Student_R2018b/Wind Controller/Grid-side Converter Controller/Current Contrl ==
  Id_ref : Inport
  Iq_ref : Inport  Port=2
  1st order Digital1 : Subsystem  mask{F0=10, Fs=Fsampling}
      mask prompts: F0 "Cut off Frequency"; Fs "Sampling Frequency"
  1st order Digital4 : Subsystem  mask{F0=10, Fs=Fsampling}
      mask prompts: F0 "Cut off Frequency"; Fs "Sampling Frequency"
  Add1 : Sum  Inputs=-+-
  Add2 : Sum  Inputs=-++
  Sum : Sum  Inputs=|+-
  Sum2 : Sum  Inputs=|+-
  Unit Delay1 : UnitDelay  SampleTime=1/Fsampling  HasFrameUpgradeWarning=on
  Unit Delay2 : UnitDelay  SampleTime=1/Fsampling  HasFrameUpgradeWarning=on
  d_coupled : Gain  Gain=Lgrid_pu_wind
  id_Ctr1 : powerlib_extras/Discrete  Control Blocks/Discrete PI Controller  Kp=0.3  Ki=200  Par_Limits=[1 -1]  Init=0  Ts=1/Fsampling
  iq_Ctr2 : powerlib_extras/Discrete  Control Blocks/Discrete PI Controller  Kp=0.3  Ki=200  Par_Limits=[1 -1]  Init=0  Ts=1/Fsampling
  q_coupled : Gain  Gain=Lgrid_pu_wind
  vd_ref : Outport
  vq_ref : Outport  Port=2
  wires:
  id_Ctr1/1 -> Add2/1
  [vd_Grid_wind] -> Add2/2
  [Iq_VSI_wind] -> d_coupled/1
  Sum/1 -> id_Ctr1/1
  iq_Ctr2/1 -> Add1/1
  [vq_Grid_wind] -> Add1/2
  [Id_VSI_wind] -> q_coupled/1
  Sum2/1 -> iq_Ctr2/1
  [Id_VSI_wind] -> Sum/2
  [Iq_VSI_wind] -> Sum2/2
  Id_ref/1 -> Sum/1
  Add2/1 -> Unit Delay1/1
  Iq_ref/1 -> Sum2/1
  Add1/1 -> Unit Delay2/1
  d_coupled/1 -> 1st order Digital4/1(in)
  q_coupled/1 -> 1st order Digital1/1(in)
  1st order Digital4/1(Out) -> Add2/3
  1st order Digital1/1(Out) -> Add1/3
  Unit Delay2/1 -> vq_ref/1
  Unit Delay1/1 -> vd_ref/1

== system MSE452_Wind_Project_Model_Student_R2018b/Wind Controller/Grid-side Converter Controller/SVM ==
  ma : Inport
  Theta : Inport  Port=2
  Pulses : Subsystem
  Sector judge : Subsystem
  Ta Tb T0 Calculation : Subsystem
  Ts : Constant  Value=1/Fs
  Zero-Order Hold : ZeroOrderHold  SampleTime=1/(2*Fs)
  Zero-Order Hold1 : ZeroOrderHold  SampleTime=1/(2*Fs)
  Gatings : Outport
  wires:
  Ta Tb T0 Calculation/3(T0) -> Pulses/4(T0)
  Ts/1 -> Ta Tb T0 Calculation/3(Ts)
  Ta Tb T0 Calculation/1(Ta1) -> Pulses/2(Ta1)
  Ta Tb T0 Calculation/2(Tb1) -> Pulses/3(Tb1)
  Sector judge/1(Sector) -> Pulses/1(Sector)
  Sector judge/2(Cal_theta) -> Ta Tb T0 Calculation/1(Cal_theta)
  Theta/1 -> Zero-Order Hold1/1
  Pulses/1(Gating) -> Gatings/1
  ma/1 -> Zero-Order Hold/1
  Zero-Order Hold/1 -> Ta Tb T0 Calculation/2(ma)
  Zero-Order Hold1/1 -> Sector judge/1(theta)

== system MSE452_Wind_Project_Model_Student_R2018b/Wind Controller/Grid-side Converter Controller/abc_dq(Current) ==
  Sin_cos : Inport
  In_Line : Inport  Port=2
  Beta : Fcn  Expr=(2/3)*(u(1)*0+u(2)*(3^0.5/2)+u(3)*(-3^0.5/2))
  Mux1 : Mux  Inputs=2
  Mux4 : Mux  Inputs=2
  Mux6 : Mux  Inputs=2
  alpha : Fcn  Expr=(2/3)*(u(1)*1+u(2)*(-1/2)+u(3)*(-1/2))
  d1 : Fcn  Expr=u(2)*u(4)+u(1)*u(3)
  q1 : Fcn  Expr=-u(2)*u(3)+u(1)*u(4)
  dq : Outport
  wires:
  Sin_cos/1 -> Mux4/2
  Beta/1 -> Mux1/1
  alpha/1 -> Mux1/2
  Mux1/1 -> Mux4/1
  In_Line/1 -> Beta/1, alpha/1
  Mux4/1 -> q1/1, d1/1
  d1/1 -> Mux6/1
  q1/1 -> Mux6/2
  Mux6/1 -> dq/1

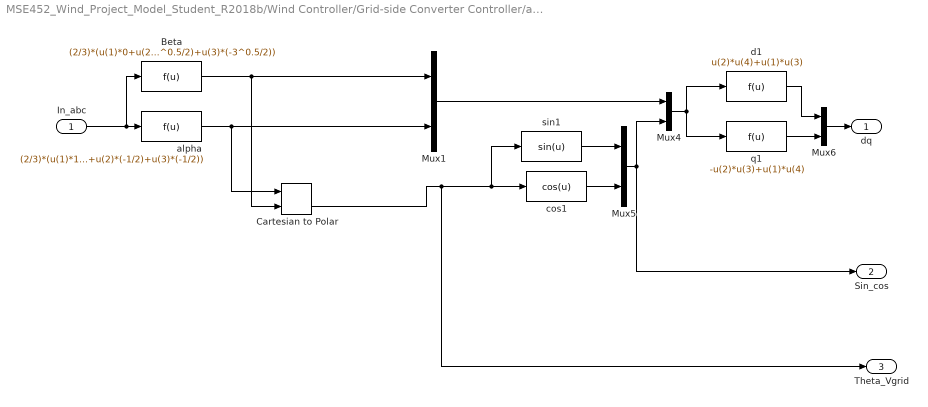
== system MSE452_Wind_Project_Model_Student_R2018b/Wind Controller/Grid-side Converter Controller/abc_dq(Voltag) ==
  In_abc : Inport
  Beta : Fcn  Expr=(2/3)*(u(1)*0+u(2)*(3^0.5/2)+u(3)*(-3^0.5/2))
  Cartesian to Polar : simulink_extras/Transformations/Cartesian to Polar
  Mux{1,4..6} (4 alike) : Mux  Inputs=2
  alpha : Fcn  Expr=(2/3)*(u(1)*1+u(2)*(-1/2)+u(3)*(-1/2))
  cos1 : Fcn  Expr=cos(u)
  d1 : Fcn  Expr=u(2)*u(4)+u(1)*u(3)
  q1 : Fcn  Expr=-u(2)*u(3)+u(1)*u(4)
  sin1 : Fcn  Expr=sin(u)
  dq : Outport
  Sin_cos : Outport  Port=2
  Theta_Vgrid : Outport  Port=3
  wires:
  Mux6/1 -> dq/1
  q1/1 -> Mux6/2
  d1/1 -> Mux6/1
  cos1/1 -> Mux5/2
  sin1/1 -> Mux5/1
  Mux4/1 -> d1/1, q1/1
  In_abc/1 -> alpha/1, Beta/1
  Mux1/1 -> Mux4/1
  alpha/1 -> Cartesian to Polar/1, Mux1/2
  Beta/1 -> Cartesian to Polar/2, Mux1/1
  Mux5/1 -> Mux4/2, Sin_cos/1
  Cartesian to Polar/2 -> cos1/1, sin1/1, Theta_Vgrid/1

== system MSE452_Wind_Project_Model_Student_R2018b/Power meter1/meter1/ voltage1/Measurements(Q28)1 ==
  InABC : Inport
  Demux : Demux  Outputs=3
  Gain1 : Gain  Gain=1/Base
  Gain2 : Gain  Gain=1/Base
  Gain3 : Gain  Gain=1/Base
  Mux : Mux  Inputs=3
  outABC : Outport  VectorParamsAs1DForOutWhenUnconnected=off
  wires:
  Mux/1 -> outABC/1
  Demux/1 -> Gain2/1
  InABC/1 -> Demux/1
  Gain2/1 -> Mux/1
  Gain1/1 -> Mux/2
  Gain3/1 -> Mux/3
  Demux/2 -> Gain1/1
  Demux/3 -> Gain3/1

== system MSE452_Wind_Project_Model_Student_R2018b/Wind Controller/Grid-side Converter Controller/Current Contrl/1st order Digital1 ==
  in : Inport
  Discrete Transfer 1Hz3 : DiscreteTransferFcn  Numerator=[1/Fs*(2*pi*F0) 1/Fs*(2*pi*F0) ]  Denominator="[((2*pi*F0)/Fs+2)  ((2*pi*F0)/Fs-2)]"  SampleTime=1/Fs
  Out : Outport
  wires:
  in/1 -> Discrete Transfer 1Hz3/1
  Discrete Transfer 1Hz3/1 -> Out/1

== system MSE452_Wind_Project_Model_Student_R2018b/Wind Controller/Grid-side Converter Controller/Current Contrl/1st order Digital4 ==
  in : Inport
  Discrete Transfer 1Hz3 : DiscreteTransferFcn  Numerator=[1/Fs*(2*pi*F0) 1/Fs*(2*pi*F0) ]  Denominator="[((2*pi*F0)/Fs+2)  ((2*pi*F0)/Fs-2)]"  SampleTime=1/Fs
  Out : Outport
  wires:
  Discrete Transfer 1Hz3/1 -> Out/1
  in/1 -> Discrete Transfer 1Hz3/1

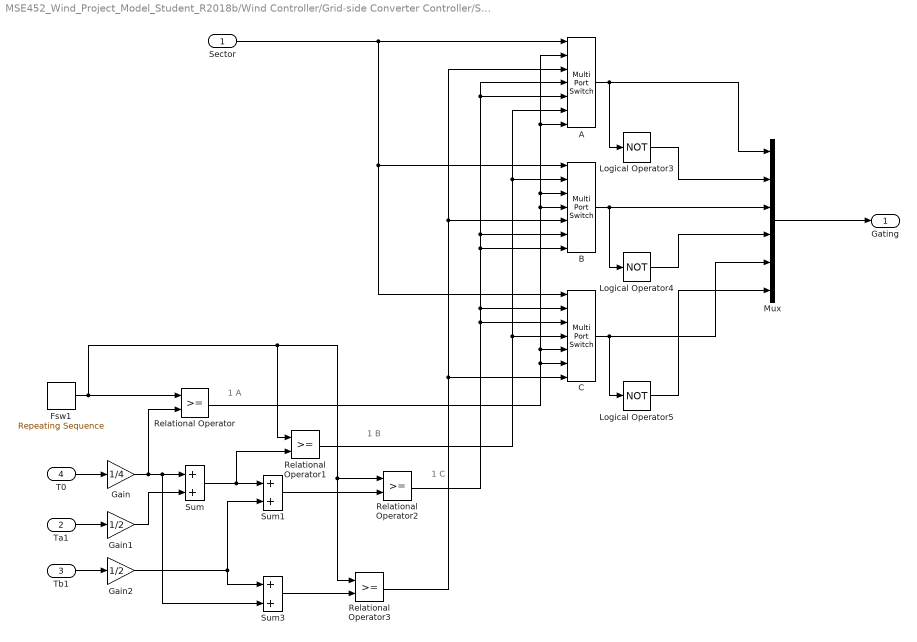
== system MSE452_Wind_Project_Model_Student_R2018b/Wind Controller/Grid-side Converter Controller/SVM/Pulses ==
  note: 1 A
  note: 1 B
  note: 1 C
  Sector : Inport
  Ta1 : Inport  Port=2
  Tb1 : Inport  Port=3
  T0 : Inport  Port=4
  A : MultiPortSwitch  Inputs=6  SaturateOnIntegerOverflow=off  InputSameDT=off
  B : MultiPortSwitch  Inputs=6  SaturateOnIntegerOverflow=off  InputSameDT=off
  C : MultiPortSwitch  Inputs=6  SaturateOnIntegerOverflow=off  InputSameDT=off
  Fsw1 : simulink/Sources/Repeating Sequence  rep_seq_t=[0 1/Fs/2 1/Fs]  rep_seq_y=[0 1/Fs/2 0]
  Gain : Gain  Gain=1/4
  Gain1 : Gain  Gain=1/2
  Gain2 : Gain  Gain=1/2
  Logical Operator3 : Logic  Operator=NOT  AllPortsSameDT=off
  Logical Operator4 : Logic  Operator=NOT  AllPortsSameDT=off
  Logical Operator5 : Logic  Operator=NOT  AllPortsSameDT=off
  Mux : Mux  Inputs=6
  Relational Operator{,1..3} (4 alike) : RelationalOperator  OutDataTypeStr=boolean  InputSameDT=off
  Sum : Sum
  Sum1 : Sum
  Sum3 : Sum
  Gating : Outport
  wires:
  T0/1 -> Gain/1
  Ta1/1 -> Gain1/1
  Tb1/1 -> Gain2/1
  Gain/1 -> Relational Operator/2, Sum/1, Sum3/2
  Gain1/1 -> Sum/2
  Gain2/1 -> Sum1/2, Sum3/1
  Sum/1 -> Sum1/1, Relational Operator1/2
  Fsw1/1 -> Relational Operator/1, Relational Operator1/1, Relational Operator2/1, Relational Operator3/1
  Sum1/1 -> Relational Operator2/2
  Sector/1 -> A/1, C/1, B/1
  A/1 -> Logical Operator3/1, Mux/1
  B/1 -> Logical Operator4/1, Mux/3
  C/1 -> Logical Operator5/1, Mux/5
  Relational Operator/1 -> A/2, A/7, B/3, B/4, C/5, C/6
  Relational Operator1/1 -> C/4, B/2, A/6
  Relational Operator2/1 -> B/7, A/4, A/5, B/6, C/2, C/3
  Mux/1 -> Gating/1
  Logical Operator3/1 -> Mux/2
  Logical Operator4/1 -> Mux/4
  Logical Operator5/1 -> Mux/6
  Sum3/1 -> Relational Operator3/2
  Relational Operator3/1 -> A/3, B/5, C/7

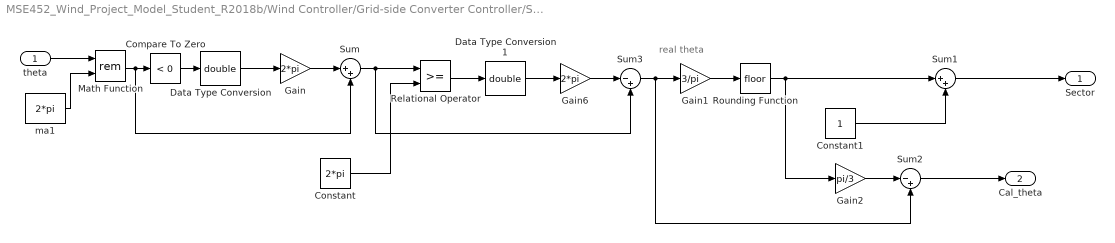
== system MSE452_Wind_Project_Model_Student_R2018b/Wind Controller/Grid-side Converter Controller/SVM/Sector judge ==
  note: real theta
  theta : Inport
  Compare To Zero : simulink/Logic and Bit Operations/Compare To Zero  relop=<  OutDataTypeStr=uint8  ZeroCross=off
  Constant : Constant  Value=2*pi
  Constant1 : Constant  OutDataTypeStr=boolean
  Data Type Conversion : DataTypeConversion  OutDataTypeStr=double  SaturateOnIntegerOverflow=off  RndMeth=Floor
  Data Type Conversion1 : DataTypeConversion  OutDataTypeStr=double  SaturateOnIntegerOverflow=off  RndMeth=Floor
  Gain : Gain  Gain=2*pi
  Gain1 : Gain  Gain=3/pi
  Gain2 : Gain  Gain=pi/3
  Gain6 : Gain  Gain=2*pi
  Math Function : Math  Operator=rem  SignedPower=on
  Relational Operator : RelationalOperator  OutDataTypeStr=boolean  InputSameDT=off
  Rounding Function : Rounding
  Sum : Sum  Inputs=|++
  Sum1 : Sum  Inputs=|++  SaturateOnIntegerOverflow=on
  Sum2 : Sum  Inputs=|-+
  Sum3 : Sum  Inputs=|-+
  ma1 : Constant  Value=2*pi
  Sector : Outport
  Cal_theta : Outport  Port=2
  wires:
  Math Function/1 -> Compare To Zero/1, Sum/2
  Compare To Zero/1 -> Data Type Conversion/1
  Data Type Conversion/1 -> Gain/1
  Gain/1 -> Sum/1
  Gain1/1 -> Rounding Function/1
  Rounding Function/1 -> Sum1/1, Gain2/1
  Sum1/1 -> Sector/1
  Constant1/1 -> Sum1/2
  Gain2/1 -> Sum2/1
  Sum2/1 -> Cal_theta/1
  Sum/1 -> Relational Operator/1, Sum3/2
  Constant/1 -> Relational Operator/2
  Relational Operator/1 -> Data Type Conversion1/1
  Data Type Conversion1/1 -> Gain6/1
  Gain6/1 -> Sum3/1
  Sum3/1 -> Gain1/1, Sum2/2
  ma1/1 -> Math Function/2
  theta/1 -> Math Function/1

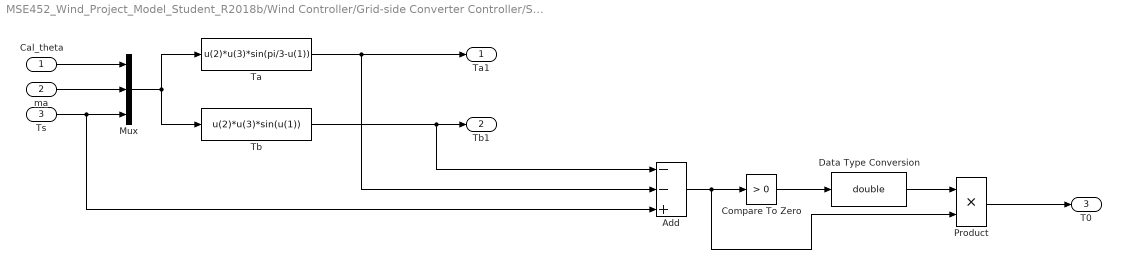
== system MSE452_Wind_Project_Model_Student_R2018b/Wind Controller/Grid-side Converter Controller/SVM/Ta Tb T0 Calculation ==
  Cal_theta : Inport
  ma : Inport  Port=2
  Ts : Inport  Port=3
  Add : Sum  Inputs=--+
  Compare To Zero : simulink/Logic and Bit Operations/Compare To Zero  relop=>  OutDataTypeStr=boolean
  Data Type Conversion : DataTypeConversion  OutDataTypeStr=double  SaturateOnIntegerOverflow=off  RndMeth=Floor
  Mux : Mux  Inputs=3
  Product : Product  RndMeth=Zero
  Ta : Fcn  Expr=u(2)*u(3)*sin(pi/3-u(1))
  Tb : Fcn  Expr=u(2)*u(3)*sin(u(1))
  Ta1 : Outport
  Tb1 : Outport  Port=2
  T0 : Outport  Port=3
  wires:
  Ts/1 -> Mux/3, Add/3
  ma/1 -> Mux/2
  Cal_theta/1 -> Mux/1
  Mux/1 -> Ta/1, Tb/1
  Ta/1 -> Add/2, Ta1/1
  Product/1 -> T0/1
  Tb/1 -> Tb1/1, Add/1
  Add/1 -> Compare To Zero/1, Product/2
  Compare To Zero/1 -> Data Type Conversion/1
  Data Type Conversion/1 -> Product/1
